simulink model "block"  (Simulink 7.7)
settings: Solver=ode45  StartTime=0.0  StopTime=0.015  RelTol=1e-3
settings Model: Creator=Johnsun  LastModifiedBy=Johnsun

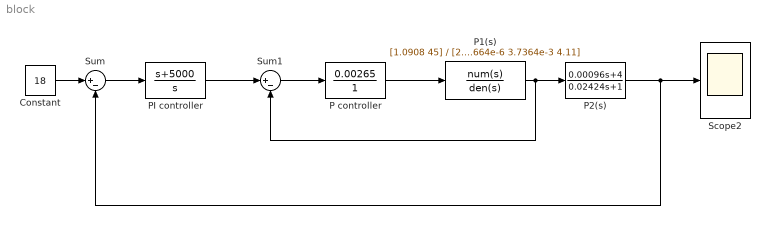
== system block ==
  Constant : Constant  Value=18
  P controller : TransferFcn  Numerator=[0.00265]  Denominator=[1]
  P1(s) : TransferFcn  Numerator=[1.0908 45]  Denominator=[2.664e-6 3.7364e-3 4.11]
  P2(s) : TransferFcn  Numerator=[0.00096 4]  Denominator=[0.02424 1]
  PI controller : TransferFcn  Numerator=[1 5000]  Denominator=[1 0]
  Scope2 : Scope
      settings: TickLabels=on  YMin=0  YMax=6.5
  Sum : Sum  Inputs=|+-
  Sum1 : Sum  Inputs=|+-
  wires:
  Sum/1 -> PI controller/1
  PI controller/1 -> Sum1/1
  Sum1/1 -> P controller/1
  P1(s)/1 -> P2(s)/1, Sum1/2
  P2(s)/1 -> Sum/2, Scope2/1
  Constant/1 -> Sum/1
  P controller/1 -> P1(s)/1
